simulink model "ConventionalVehicle"  (R2018a)
settings: Solver=VariableStepAuto  StartTime=0.0  StopTime=TimeUS06  FixedStep=.1  MaxStep=1  RelTol=1e-3  AbsTol=1  EnableMultiTasking=on
PostLoadFcn:
  | addpath('ImagesConventional')
  | 
  | ConventionalDir = pwd;
  | 
  | cd ..\;
  | SimulinkDir = pwd;
  | addpath(SimulinkDir);
  | 
  | cd(ConventionalDir);
model workspace (MAT data in the model file):
  DownShiftSpeeds = [11.05  11.05  11.05  11.05  11.05  11.05  11.05  11.05  11.05  11.05  11.05  11.05  19.55  25.5  31.45  35.7  35.7; 18.7  18.7  18.7  18.7  19.125  20.48636  21.33636  23.375  27.28636  30.26136  33.827365  38.76136  46.072635  56.1  64.6  73.1  73.1; 28.9  28.9  28.9  28.9  28.9  30.51364  34.51136  41.56364  47.68636  53.377365  58.477365  65.622635  73.525  81.26136  88.48636  115.6  115.6; 38.675  38.675  38.675  38.675  39.43864  42.41364  47.68636  56.43864  65.11136  72.927365  80.497635  90.01364  100.81136  110.672635  122.4  153  153; 51.425  51.425  51.425  51.425  51.76364  55.077365  62.38864  72.422635  83.3  102  136  425  425  425  425  425  425]
  DrCycles.C505 = [0 1 2 3 4 5 6 7 8 9 10 11 ... (1012 elements, 506x2)]
  DrCycles.FTP = [0 1 2 3 4 5 6 7 8 9 10 11 ... (4956 elements, 2478x2)]
  DrCycles.UDDS = [0 1 2 3 4 5 6 7 8 9 10 11 ... (2746 elements, 1373x2)]
  DrCycles.HWFET = [0 1 2 3 4 5 6 7 8 9 10 11 ... (1532 elements, 766x2)]
  DrCycles.US06 = [0 1 2 3 4 5 6 7 8 9 10 11 ... (1194 elements, 597x2)]
  DrCycles.US06City = [0 1 2 3 4 5 6 7 8 9 10 11 ... (466 elements, 233x2)]
  DrCycles.US06Hwy = [0 1 2 3 4 5 6 7 8 9 10 11 ... (742 elements, 371x2)]
  FD = 3.4
  G1 = 4.47
  G2 = 2.47
  G3 = 1.47
  G4 = 1
  G5 = 0.8
  G6 = 0.65
  MDL.EngineModel.BMEPtbl = [0  0; 1000  800000; 1200  900000; 1800  1000000; 2400  1100000; 3200  1200000; 3600  1200000; 4000  1200000; 4400  1200000; 4800  1200000; 5600  1100000; 6000  1000000]
  MDL.EngineModel.Vdisp = 0.0053
  MDL.EngineModel.MaxPwr = 280000
  MDL.EngineModel.MaxTrq = 500
  MDL.EngineModel.EtaT = 0.46
  MDL.EngineModel.fmep0 = 140000
  MDL.EngineModel.fmep1 = 15.2
  MDL.EngineModel.C2 = 1e-06
  MDL.EngineModel.LHV = 42120000
  MDL.EngineModel.FuelEnergyDensByVol = 33700
  MDL.EngineModel.AccyLoad = 600
  MDL.EngineModel.MinTrq = 8
  MDL.DrivelineModel.C0 = 8
  MDL.DrivelineModel.C1 = 10
  MDL.DrivelineModel.C2 = 4
  MDL.DrivelineModel.Ftr_max = 5000
  PedalPositions = [0 6.2485 12.4969 18.7454 24.9939 31.2424 37.4908 43.7393 49.9878 56.2363 62.4847 68.7332 74.9817 81.2302 87.4786 93.7271 99.9756]
  TimeHWFET = 765
  TimeUDDS = 1372
  TimeUS06 = 596
  UpShiftSpeeds = [12.75  12.75  12.75  12.75  12.75  12.75  15.552365  17.08636  18.7  20.227365  23.46136  27.625  31.702365  36.63636  42.5  42.5  42.5; 20.997635  20.997635  20.997635  20.997635  21.927365  24.902365  28.727365  31.78864  35.275  39.697635  46.41136  51.85  59.672635  67.48864  78.2  78.2  78.2; 31.45  31.45  31.45  31.45  34.172635  41.052365  47.175  52.952365  59.5  68  76.5  85  93.5  106.25  119.85  119.85  119.85; 42.16136  42.16136  42.16136  43.947635  47.002365  54.31364  63.325  71.227365  79.222635  88.06136  98.852365  109.052365  118.402365  128.86136  157.25  157.25  157.25; 55.58864  55.58864  55.58864  58.052365  61.53864  72.077365  85.51136  96.81364  255  255  255  255  255  255  255  255  255]
  aeroDragCoeff = 0.38
  airDensity = 1.23
  frontArea = 2.1
  gravity = 9.81
  inclinationAngle = 0
  inertialMassVeh = 2392
  massVeh = 2300
  rollingResistCoeff = 0.01
  wheelRadius = 0.35
libraries: Driver_Glider_Library x2, simulink x1
CloseFcn:
  | rmpath(SimulinkDir);
  | rmpath('ImagesConventional')
  | clear ConventionalDir SimulinkDir;
settings Model: Creator=David  LastModifiedBy=emarquez
settings SolverCC: AutoScaleAbsTol=off
settings DataIOCC: ExternalInput=DriveCycle  SaveFormat=Array  SignalLoggingSaveFormat=ModelDataLogs
settings OptimizationCC: ExpressionDepthLimit=2147483647  LifeSpan=inf
settings DebuggingCC: UnderspecifiedInitializationDetection=Classic  MergeDetectMultiDrivingBlocksExec=none  SolverPrmCheckMsg=warning  FcnCallInpInsideContextMsg=warning  StateNameClashWarn=warning  SFUnexpectedBacktrackingDiag=warning  SFNoUnconditionalDefaultTransitionDiag=warning  SFExecutionAtInitializationDiag=none
settings HardwareCC: ProdBitPerPointer=32  ProdBitPerSizeT=32  ProdBitPerPtrDiffT=32  ProdLargestAtomicFloat=None  ProdIntDivRoundTo=Undefined  ProdEndianess=Unspecified  ProdWordSize=32  ProdHWDeviceType=32-bit Generic
settings ModelReferenceCC: PropagateSignalLabelsOutOfModel=off
settings CodeAppCC: StateflowObjectComments=on
settings GRTTargetCC: TargetLangStandard=C89/C90 (ANSI)  GeneratePreprocessorConditionals=Disable all  CombineOutputUpdateFcns=off  GRTInterface=on
settings ConfigComp: CovMetricSettings=dw  CovHtmlReporting=on  CovSaveCumulativeToWorkspaceVar=on  CovSaveSingleToWorkspaceVar=on  CovExternalEMLEnable=off  CovSFcnEnable=off

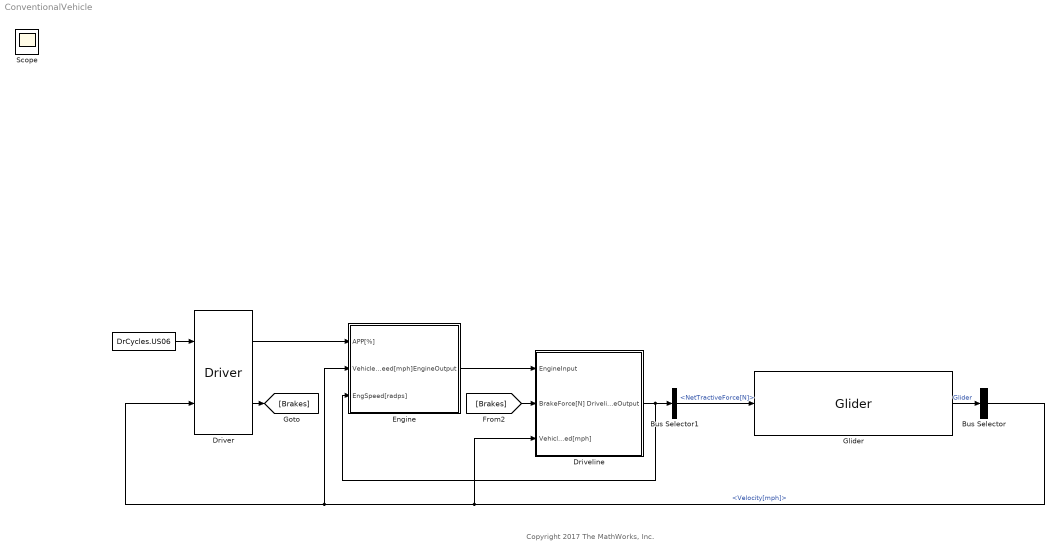
== system ConventionalVehicle ==
  note: Copyright 2017 The MathWorks, Inc.
  " " : FromWorkspace  Tag=DriveCycle  VariableName=DrCycles.US06  SampleTime=0
  Bus Selector : BusSelector  OutputSignals=Velocity[mph]
  Bus Selector1 : BusSelector  OutputSignals=NetTractiveForce[N]
  Driveline : Subsystem
      mask Display: image('driveline.jpg');
  Driver : Driver_Glider_Library/Driver  SystemSampleTime=-1
  Engine : Subsystem
      mask Display: image('engine.jpg');
  Glider : Driver_Glider_Library/Glider  SystemSampleTime=-1
  Scope : Scope
  wires:
  Glider/1 -> Bus Selector/1  "Glider"
  Driver/1 -> Engine/1(APP[%])
  Engine/1(EngineOutput) -> Driveline/1(EngineInput)
  Driveline/1(DrivelineOutput) -> Bus Selector1/1, Engine/3(EngSpeed[radps])
  " "/1 -> Driver/1
  Driver/2 -> [Brakes]
  [Brakes] -> Driveline/2(BrakeForce[N])
  Bus Selector/1 -> Driver/2, Engine/2(VehicleSpeed[mph]), Driveline/3(VehicleSpeed[mph])  "<Velocity[mph]>"
  Bus Selector1/1 -> Glider/1  "<NetTractiveForce[N]>"

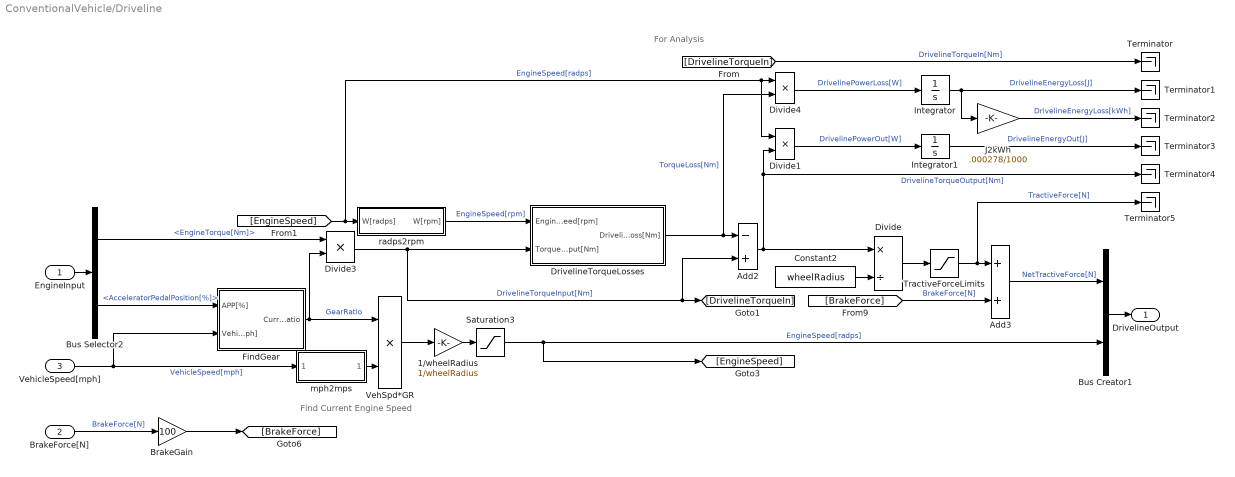
== system ConventionalVehicle/Driveline ==
  note: For Analysis
  note: Find Current Engine Speed
  EngineInput : Inport
  BrakeForce[N] : Inport  Port=2
  VehicleSpeed[mph] : Inport  Port=3
  1/wheelRadius : Gain  Gain=1/wheelRadius
  Add2 : Sum  Inputs=-+
  Add3 : Sum
  BrakeGain : Gain  Gain=100
  Bus Creator1 : BusCreator  Inputs=2
  Bus Selector2 : BusSelector  OutputSignals=EngineTorque[Nm],AcceleratorPedalPosition[%]
  Constant2 : Constant  Value=wheelRadius
  Divide : Product  Inputs=*/
  Divide1 : Product  Inputs=**
  Divide3 : Product  Inputs=**
  Divide4 : Product  Inputs=**
  DrivelineTorqueLosses : Subsystem
  FindGear : Subsystem
  Integrator : Integrator
  Integrator1 : Integrator
  J2kWh : Gain  Gain=.000278/1000
  Saturation3 : Saturate  UpperLimit=inf  LowerLimit=0.001  ZeroCross=off
  Terminator{,1..5} (6 alike) : Terminator
  TractiveForceLimits : Saturate  UpperLimit=MDL.DrivelineModel.Ftr_max  LowerLimit=0  ZeroCross=off
  VehSpd*GR : Product  Inputs=**
  mph2mps : Subsystem
  radps2rpm : Subsystem
  DrivelineOutput : Outport
  wires:
  Add2/1 -> Divide/1, Divide1/2, Terminator4/1  "DrivelineTorqueOutput[Nm]"
  Divide/1 -> TractiveForceLimits/1
  [BrakeForce] -> Add3/2  "BrakeForce[N]"
  TractiveForceLimits/1 -> Terminator5/1, Add3/1  "TractiveForce[N]"
  EngineInput/1 -> Bus Selector2/1
  Add3/1 -> Bus Creator1/1  "NetTractiveForce[N]"
  1/wheelRadius/1 -> Saturation3/1
  Saturation3/1 -> [EngineSpeed], Bus Creator1/2  "EngineSpeed[radps]"
  VehSpd*GR/1 -> 1/wheelRadius/1
  FindGear/1(CurrentGearRatio) -> Divide3/2, VehSpd*GR/1  "GearRatio"
  Constant2/1 -> Divide/2
  Bus Selector2/1 -> Divide3/1  "<EngineTorque[Nm]>"
  Divide3/1 -> Add2/2, [DrivelineTorqueIn], DrivelineTorqueLosses/2(TorqueInput[Nm])  "DrivelineTorqueInput[Nm]"
  Divide4/1 -> Integrator/1  "DrivelinePowerLoss[W]"
  [EngineSpeed] -> Divide1/1, Divide4/1, radps2rpm/1(W[radps])  "EngineSpeed[radps]"
  Divide1/1 -> Integrator1/1  "DrivelinePowerOut[W]"
  Integrator1/1 -> Terminator3/1  "DrivelineEnergyOut[J]"
  J2kWh/1 -> Terminator2/1  "DrivelineEnergyLoss[kWh]"
  Integrator/1 -> J2kWh/1, Terminator1/1  "DrivelineEnergyLoss[J]"
  Bus Selector2/2 -> FindGear/1(APP[%])  "<AcceleratorPedalPosition[%]>"
  DrivelineTorqueLosses/1(DrivelineTorqueLoss[Nm]) -> Divide4/2, Add2/1  "TorqueLoss[Nm]"
  radps2rpm/1(W[rpm]) -> DrivelineTorqueLosses/1(EngineSpeed[rpm])  "EngineSpeed[rpm]"
  Bus Creator1/1 -> DrivelineOutput/1
  [DrivelineTorqueIn] -> Terminator/1  "DrivelineTorqueIn[Nm]"
  BrakeForce[N]/1 -> BrakeGain/1  "BrakeForce[N]"
  VehicleSpeed[mph]/1 -> mph2mps/1(V[mph]), FindGear/2(VehicleSpeed[mph])  "VehicleSpeed[mph]"
  BrakeGain/1 -> [BrakeForce]
  mph2mps/1(V[mps]) -> VehSpd*GR/2

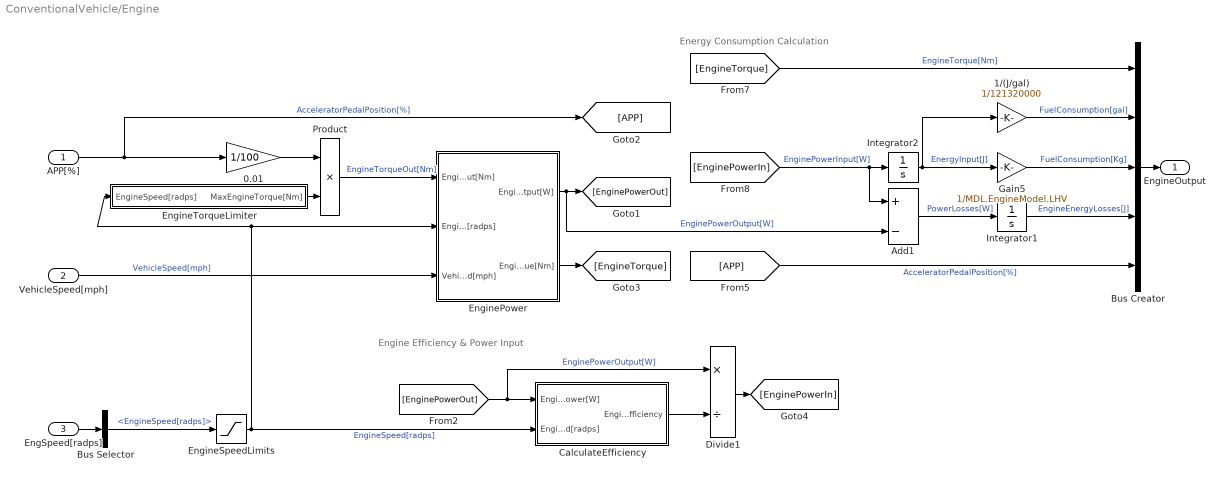
== system ConventionalVehicle/Engine ==
  note: Engine Efficiency & Power Input
  note: Energy Consumption Calculation
  APP[%] : Inport
  VehicleSpeed[mph] : Inport  Port=2
  EngSpeed[radps] : Inport  Port=3
  0.01 : Gain  Gain=1/100
  1/(J/gal) : Gain  Gain=1/121320000
  Add1 : Sum  Inputs=+-
  Bus Creator : BusCreator  Inputs=5
  Bus Selector : BusSelector  OutputSignals=EngineSpeed[radps]
  CalculateEfficiency : Subsystem
  Divide1 : Product  Inputs=*/
  EnginePower : Subsystem
  EngineSpeedLimits : Saturate  UpperLimit=940  LowerLimit=84
  EngineTorqueLimiter : Subsystem
  Gain5 : Gain  Gain=1/MDL.EngineModel.LHV
      settings: AttributesFormatString=%<Gain>
  Integrator1 : Integrator
  Integrator2 : Integrator
  Product : Product  RndMeth=Zero
  EngineOutput : Outport
  wires:
  APP[%]/1 -> [APP], 0.01/1  "AcceleratorPedalPosition[%]"
  0.01/1 -> Product/1
  Integrator2/1 -> Gain5/1, 1/(J/gal)/1  "EnergyInput[J]"
  Bus Creator/1 -> EngineOutput/1
  1/(J/gal)/1 -> Bus Creator/2  "FuelConsumption[gal]"
  Integrator1/1 -> Bus Creator/4  "EngineEnergyLosses[J]"
  Gain5/1 -> Bus Creator/3  "FuelConsumption[Kg]"
  EngSpeed[radps]/1 -> Bus Selector/1
  CalculateEfficiency/1(EngineEfficiency) -> Divide1/2
  Add1/1 -> Integrator1/1  "PowerLosses[W]"
  [APP] -> Bus Creator/5  "AcceleratorPedalPosition[%]"
  EngineTorqueLimiter/1(MaxEngineTorque[Nm]) -> Product/2
  Product/1 -> EnginePower/1(EngineTorqueOut[Nm])  "EngineTorqueOut[Nm]"
  EngineSpeedLimits/1 -> EnginePower/2(EngineSpeed[radps]), EngineTorqueLimiter/1(EngineSpeed[radps]), CalculateEfficiency/2("EngineSpeed[radps] ")  "EngineSpeed[radps]"
  VehicleSpeed[mph]/1 -> EnginePower/3(VehicleSpeed[mph])  "VehicleSpeed[mph]"
  Bus Selector/1 -> EngineSpeedLimits/1  "<EngineSpeed[radps]>"
  [EnginePowerOut] -> Divide1/1, CalculateEfficiency/1(EnginePower[W])  "EnginePowerOutput[W]"
  EnginePower/1(EnginePowerOutput[W]) -> [EnginePowerOut], Add1/2  "EnginePowerOutput[W]"
  EnginePower/2(EngineTorque[Nm]) -> [EngineTorque]
  [EngineTorque] -> Bus Creator/1  "EngineTorque[Nm]"
  Divide1/1 -> [EnginePowerIn]
  [EnginePowerIn] -> Add1/1, Integrator2/1  "EnginePowerInput[W]"

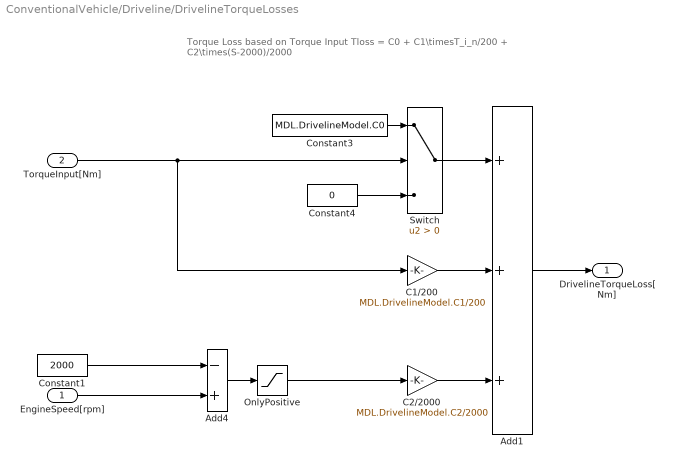
== system ConventionalVehicle/Driveline/DrivelineTorqueLosses ==
  note: Torque Loss based on Torque Input
      | Tloss = C0 + C1\timesT_i_n/200 + C2\times(S-2000)/2000
  EngineSpeed[rpm] : Inport
  TorqueInput[Nm] : Inport  Port=2
  Add1 : Sum  Inputs=+++
  Add4 : Sum  Inputs=-+
  C1/200 : Gain  Gain=MDL.DrivelineModel.C1/200
      settings: AttributesFormatString=%<Gain>
  C2/2000 : Gain  Gain=MDL.DrivelineModel.C2/2000
      settings: AttributesFormatString=%<Gain>
  Constant1 : Constant  Value=2000
  Constant3 : Constant  Value=MDL.DrivelineModel.C0
  Constant4 : Constant  Value=0
  OnlyPositive : Saturate  UpperLimit=inf  LowerLimit=0
  Switch : Switch  Criteria=u2 > Threshold  ZeroCross=off
  DrivelineTorqueLoss[Nm] : Outport
  wires:
  TorqueInput[Nm]/1 -> C1/200/1, Switch/2
  Constant3/1 -> Switch/1
  C1/200/1 -> Add1/2
  Add4/1 -> OnlyPositive/1
  Constant1/1 -> Add4/1
  C2/2000/1 -> Add1/3
  Add1/1 -> DrivelineTorqueLoss[Nm]/1
  Switch/1 -> Add1/1
  OnlyPositive/1 -> C2/2000/1
  Constant4/1 -> Switch/3
  EngineSpeed[rpm]/1 -> Add4/2

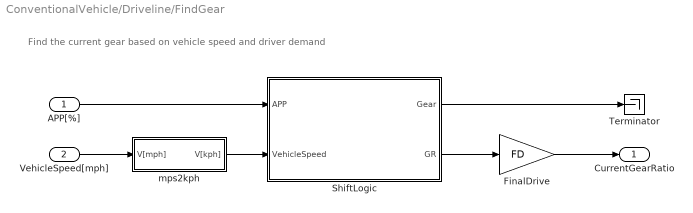
== system ConventionalVehicle/Driveline/FindGear ==
  note: Find the current gear based on vehicle speed and driver demand
  APP[%] : Inport
  VehicleSpeed[mph] : Inport  Port=2
  FinalDrive : Gain  Gain=FD
  ShiftLogic : Stateflow chart  TreatAsAtomicUnit=on
  Terminator : Terminator
  mps2kph : Subsystem
  CurrentGearRatio : Outport
  wires:
  VehicleSpeed[mph]/1 -> mps2kph/1(V[mph])
  ShiftLogic/1(Gear) -> Terminator/1
  ShiftLogic/2(GR) -> FinalDrive/1
  FinalDrive/1 -> CurrentGearRatio/1
  mps2kph/1(V[kph]) -> ShiftLogic/2(VehicleSpeed)
  APP[%]/1 -> ShiftLogic/1(APP)

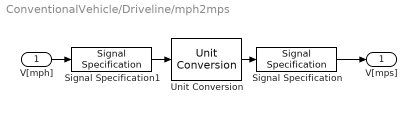
== system ConventionalVehicle/Driveline/mph2mps ==
  V[mph] : Inport
  Signal Specification : SignalSpecification  Unit=m/s
  Signal Specification1 : SignalSpecification  Unit=mph
  Unit Conversion : UnitConversion
  V[mps] : Outport
  wires:
  V[mph]/1 -> Signal Specification1/1
  Unit Conversion/1 -> Signal Specification/1
  Signal Specification1/1 -> Unit Conversion/1
  Signal Specification/1 -> V[mps]/1

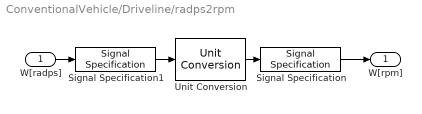
== system ConventionalVehicle/Driveline/radps2rpm ==
  W[radps] : Inport
  Signal Specification : SignalSpecification  Unit=rpm
  Signal Specification1 : SignalSpecification  Unit=rad/s
  Unit Conversion : UnitConversion
  W[rpm] : Outport
  wires:
  W[radps]/1 -> Signal Specification1/1
  Unit Conversion/1 -> Signal Specification/1
  Signal Specification1/1 -> Unit Conversion/1
  Signal Specification/1 -> W[rpm]/1

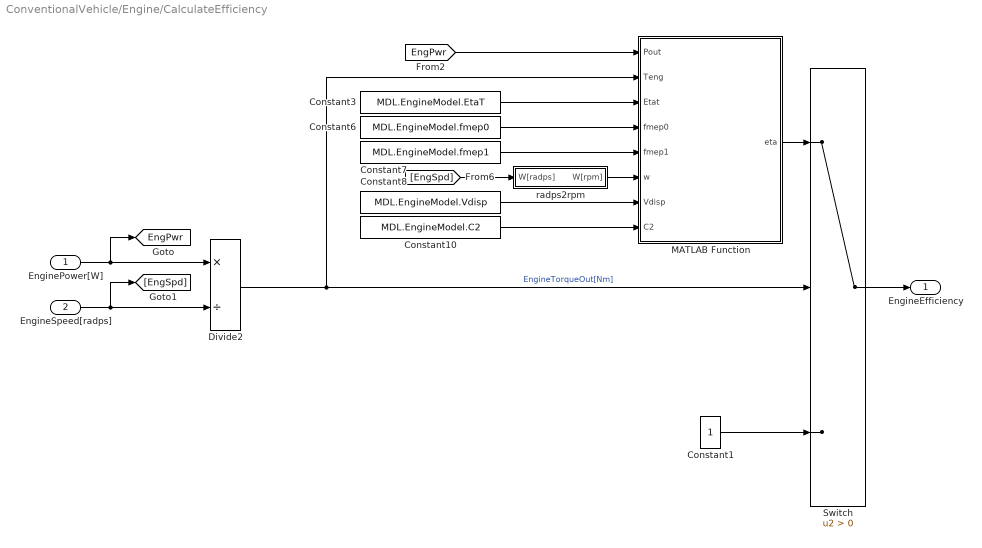
== system ConventionalVehicle/Engine/CalculateEfficiency ==
  EnginePower[W] : Inport
  "EngineSpeed[radps] " : Inport  Port=2
  Constant1 : Constant
  Constant10 : Constant  Value=MDL.EngineModel.C2
  Constant3 : Constant  Value=MDL.EngineModel.EtaT
  Constant6 : Constant  Value=MDL.EngineModel.fmep0
  Constant7 : Constant  Value=MDL.EngineModel.fmep1
  Constant8 : Constant  Value=MDL.EngineModel.Vdisp
  "Divide2  " : Product  Inputs=*/
  MATLAB Function : MATLAB Function  TreatAsAtomicUnit=on
  Switch : Switch  Criteria=u2 > Threshold  ZeroCross=off
  radps2rpm : Subsystem
  EngineEfficiency : Outport
  tag scope: EngPwr=global
  wires:
  "EngineSpeed[radps] "/1 -> [EngSpd], "Divide2  "/2
  "Divide2  "/1 -> Switch/2, MATLAB Function/2(Teng)  "EngineTorqueOut[Nm]"
  EnginePower[W]/1 -> [EngPwr], "Divide2  "/1
  Switch/1 -> EngineEfficiency/1
  Constant1/1 -> Switch/3
  [EngPwr] -> MATLAB Function/1(Pout)
  Constant3/1 -> MATLAB Function/3(Etat)
  Constant6/1 -> MATLAB Function/4(fmep0)
  Constant7/1 -> MATLAB Function/5(fmep1)
  Constant8/1 -> MATLAB Function/7(Vdisp)
  Constant10/1 -> MATLAB Function/8(C2)
  [EngSpd] -> radps2rpm/1(W[radps])
  MATLAB Function/1(eta) -> Switch/1
  radps2rpm/1(W[rpm]) -> MATLAB Function/6(w)

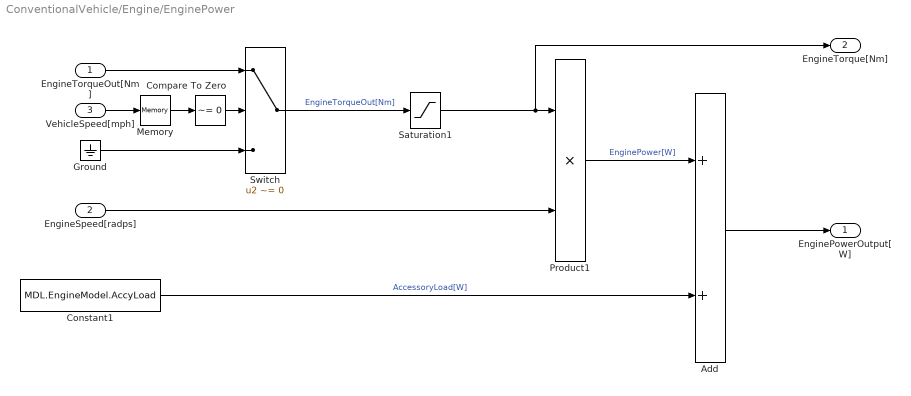
== system ConventionalVehicle/Engine/EnginePower ==
  EngineTorqueOut[Nm] : Inport
  EngineSpeed[radps] : Inport  Port=2
  VehicleSpeed[mph] : Inport  Port=3
  Add : Sum
  Compare To Zero : simulink/Logic and Bit Operations/Compare To Zero  relop=~=  OutDataTypeStr=boolean
  Constant1 : Constant  Value=MDL.EngineModel.AccyLoad
  Ground : Ground
  Memory : Memory
  Product1 : Product  RndMeth=Zero
  Saturation1 : Saturate  UpperLimit=MDL.EngineModel.MaxTrq  LowerLimit=8
  Switch : Switch  Criteria=u2 ~= 0  Threshold=.5
  EnginePowerOutput[W] : Outport
  EngineTorque[Nm] : Outport  Port=2
  wires:
  Constant1/1 -> Add/2  "AccessoryLoad[W]"
  Add/1 -> EnginePowerOutput[W]/1
  Saturation1/1 -> EngineTorque[Nm]/1, Product1/1
  Switch/1 -> Saturation1/1  "EngineTorqueOut[Nm]"
  Product1/1 -> Add/1  "EnginePower[W]"
  Memory/1 -> Compare To Zero/1
  EngineSpeed[radps]/1 -> Product1/2
  VehicleSpeed[mph]/1 -> Memory/1
  EngineTorqueOut[Nm]/1 -> Switch/1
  Ground/1 -> Switch/3
  Compare To Zero/1 -> Switch/2

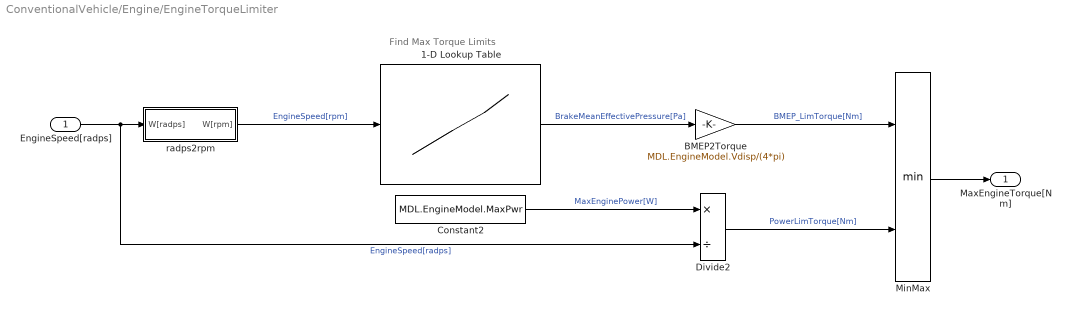
== system ConventionalVehicle/Engine/EngineTorqueLimiter ==
  note: Find Max Torque Limits
  EngineSpeed[radps] : Inport
  1-D Lookup Table : Lookup_n-D  NumberOfTableDimensions=1  BreakpointsForDimension1=MDL.EngineModel.BMEPtbl(:,1)  BreakpointsForDimension2=[1:length(MDL.EngineModel.TrqTbl)]  Table=MDL.EngineModel.BMEPtbl(:,2)  RndMeth=Simplest  InputSameDT=on
  BMEP2Torque : Gain  Gain=MDL.EngineModel.Vdisp/(4*pi)
      settings: AttributesFormatString=%<Gain>
  Constant2 : Constant  Value=MDL.EngineModel.MaxPwr
  Divide2 : Product  Inputs=*/
  MinMax : MinMax  Inputs=2
  radps2rpm : Subsystem
  MaxEngineTorque[Nm] : Outport
  wires:
  Constant2/1 -> Divide2/1  "MaxEnginePower[W]"
  EngineSpeed[radps]/1 -> radps2rpm/1(W[radps]), Divide2/2  "EngineSpeed[radps]"
  1-D Lookup Table/1 -> BMEP2Torque/1  "BrakeMeanEffectivePressure[Pa]"
  MinMax/1 -> MaxEngineTorque[Nm]/1
  Divide2/1 -> MinMax/2  "PowerLimTorque[Nm]"
  BMEP2Torque/1 -> MinMax/1  "BMEP_LimTorque[Nm]"
  radps2rpm/1(W[rpm]) -> 1-D Lookup Table/1  "EngineSpeed[rpm]"

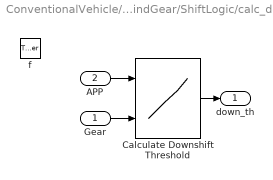
== system ConventionalVehicle/Driveline/FindGear/ShiftLogic/calc_down ==
  Gear : Inport
  APP : Inport  Port=2
  f : TriggerPort  TriggerType=function-call  VariantControl=Variant
      settings: CopyFcn=Stateflow.SLINSF.SimulinkMan.removeBlockPreDeleteFcn  PreDeleteFcn=Stateflow.SLINSF.SimulinkMan.unsafePredeleteFcn
  Calculate Downshift Threshold : Lookup2D  RowIndex=PedalPositions  ColumnIndex=[2,3,4,5,6]  Table=DownShiftSpeeds'  LookUpMeth=Interpolation-Use End Values
  down_th : Outport
  wires:
  Calculate Downshift Threshold/1 -> down_th/1
  Gear/1 -> Calculate Downshift Threshold/2
  APP/1 -> Calculate Downshift Threshold/1

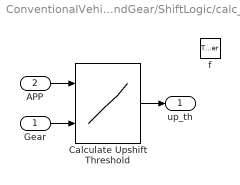
== system ConventionalVehicle/Driveline/FindGear/ShiftLogic/calc_up ==
  Gear : Inport
  APP : Inport  Port=2
  f : TriggerPort  TriggerType=function-call  VariantControl=Variant
      settings: CopyFcn=Stateflow.SLINSF.SimulinkMan.removeBlockPreDeleteFcn  PreDeleteFcn=Stateflow.SLINSF.SimulinkMan.unsafePredeleteFcn
  Calculate Upshift Threshold : Lookup2D  RowIndex=PedalPositions  ColumnIndex=[1,2,3,4,5]  Table=UpShiftSpeeds'  LookUpMeth=Interpolation-Use End Values
  up_th : Outport
  wires:
  Calculate Upshift Threshold/1 -> up_th/1
  APP/1 -> Calculate Upshift Threshold/1
  Gear/1 -> Calculate Upshift Threshold/2

== system ConventionalVehicle/Driveline/FindGear/mps2kph ==
  V[mph] : Inport
  Signal Specification : SignalSpecification  Unit=km/hr
  Signal Specification1 : SignalSpecification  Unit=mph
  Unit Conversion : UnitConversion
  V[kph] : Outport
  wires:
  V[mph]/1 -> Signal Specification1/1
  Unit Conversion/1 -> Signal Specification/1
  Signal Specification1/1 -> Unit Conversion/1
  Signal Specification/1 -> V[kph]/1

== system ConventionalVehicle/Engine/CalculateEfficiency/radps2rpm ==
  W[radps] : Inport
  Signal Specification : SignalSpecification  Unit=rpm
  Signal Specification1 : SignalSpecification  Unit=rad/s
  Unit Conversion : UnitConversion
  W[rpm] : Outport
  wires:
  W[radps]/1 -> Signal Specification1/1
  Unit Conversion/1 -> Signal Specification/1
  Signal Specification1/1 -> Unit Conversion/1
  Signal Specification/1 -> W[rpm]/1

== system ConventionalVehicle/Engine/EngineTorqueLimiter/radps2rpm ==
  W[radps] : Inport
  Signal Specification : SignalSpecification  Unit=rpm
  Signal Specification1 : SignalSpecification  Unit=rad/s
  Unit Conversion : UnitConversion
  W[rpm] : Outport
  wires:
  W[radps]/1 -> Signal Specification1/1
  Unit Conversion/1 -> Signal Specification/1
  Signal Specification1/1 -> Unit Conversion/1
  Signal Specification/1 -> W[rpm]/1

== stateflow chart ConventionalVehicle/Driveline/FindGear/ShiftLogic ==
  settings: updateMethod=DISCRETE  sampleTime=0.1
  state gear_state [parallel]
    settings: executionOrder=1
    state first
      entry:
      Gear = 1;
      GR = G1;
    state second
      entry:
      Gear = 2;
      GR = G2;
    state third
      entry:
      Gear = 3;
      GR = G3;
    state fourth
      entry:
      Gear = 4;
      GR = G4;
    state fifth
      entry:
      Gear = 5;
      GR = G5;
    state sixth
      entry:
      Gear = 6;
      GR = G6;
    (default) -> first
    second -> third [order 1] : UP
    first -> second : UP
    fourth -> fifth [order 1] : UP
    fifth -> sixth [order 1] : UP
    third -> fourth [order 1] : UP
    third -> second [order 2] : DOWN
    second -> first [order 2] : DOWN
    fifth -> fourth [order 2] : DOWN
    fourth -> third [order 2] : DOWN
    sixth -> fifth : DOWN
  state selection_state [parallel]
    du:[up_th]=calc_up(Gear,APP);
    du:[down_th]=calc_down(Gear,APP);
    settings: executionOrder=2
    state steady_state
    state upshifting
    state downshifting
    (default) -> steady_state
    steady_state -> upshifting [order 1] : [VehicleSpeed > up_th]
    steady_state -> downshifting [order 2] : [VehicleSpeed < down_th && Gear > 1]
    downshifting -> steady_state [order 1] : after(1,tick)
        | [VehicleSpeed <= down_th]
        | {gear_state.DOWN;}
    downshifting -> steady_state [order 2] : [VehicleSpeed > down_th]
    upshifting -> steady_state [order 1] : after(1,tick)
        | [VehicleSpeed >= up_th]
        | {gear_state.UP;}
    upshifting -> steady_state [order 2] : [VehicleSpeed < up_th]
  state up_th = calc_up(Gear,APP) [function]
  state down_th = calc_down(Gear,APP) [function]
  data: Gear function_input; APP function_input; up_th function_output; Gear function_input; APP function_input; down_th function_output; APP input double [0..100]; VehicleSpeed input double; Gear output double; down_th local double; up_th local double; GR output double; G1 parameter double; G2 parameter double; G3 parameter double; G4 parameter double; G5 parameter double; G6 parameter double
  events: DOWN local EITHER_EDGE_EVENT; UP local EITHER_EDGE_EVENT

== matlab function ConventionalVehicle/Engine/CalculateEfficiency/MATLAB Function ==
  data: Pout input; eta output; Teng input; Etat input; fmep0 input; fmep1 input; w input; Vdisp input; C2 input
function eta = EngineEfficiency(Pout,Teng,Etat,fmep0,fmep1,w,Vdisp,C2)
%#codegen

eta = Pout/(Pout/(Etat/(1+(fmep0+fmep1*w)/(4*pi*Teng/Vdisp)))+C2*Pout^2);
